simulink library "est_estimator_lib_wState_lib"  (R2016b)
settings: Solver=ode45  StartTime=0.0  StopTime=10.0  RelTol=1e-3  EnableMultiTasking=on
values from neighbouring files (symbols this model uses):
  ase_accel_fixed_bias = single([0 0 0])    [ase_augmented_state_estimator_init.m]    (also in ase_hw_data_test.m = single([-0.1425    0.0852   -9.8201]))
  ase_gyro_fixed_bias = single([0 0 0])    [ase_augmented_state_estimator_init.m]    (also in ase_hw_data_test.m = single(1e-3 * [-1.0787    0.00   0.4470]))
  ase_ml_num_features = Simulink.Parameter(int32(50))    [ase_augmented_state_estimator_init.m]
  ase_of_num_aug = Simulink.Parameter(int32(16))    [ase_augmented_state_estimator_init.m]
  ase_of_num_features = Simulink.Parameter(int32(50))    [ase_augmented_state_estimator_init.m]
  ase_ts = astrobee_fsw_step_size    [ase_augmented_state_estimator_init.m]
undefined symbols (not defined in the file or in its folder): astrobee_fsw_step_size, fam_impeller_speeds, tun_abp_quat_body2imu, tun_ase_gravity_accel, tun_ase_gravity_removal, tun_grav_hp_den, tun_grav_hp_enable_f, tun_grav_hp_num, tun_ic_cov_pos, tun_ic_cov_quat
libraries: simulink x10, math_utils x3, delay_ic_lib x1, camera_update_lib x1, output_prep_lib x1, predictor_lib x1, state_manager_lib x1
settings Model: Creator=jfusco1  LastModifiedBy=jfusco1
settings DataIOCC: LimitDataPoints=on  SaveFormat=Array
settings OptimizationCC: LifeSpan=inf
settings DebuggingCC: AllowSymbolicDim=off  SFUnexpectedBacktrackingDiag=warning  SFNoUnconditionalDefaultTransitionDiag=warning  SFExecutionAtInitializationDiag=none
settings HardwareCC: ProdBitPerPointer=32  ProdBitPerSizeT=32  ProdBitPerPtrDiffT=32  ProdLargestAtomicFloat=None  ProdIntDivRoundTo=Undefined  ProdEndianess=Unspecified  ProdWordSize=32  ProdHWDeviceType=32-bit Generic
settings ModelReferenceCC: PropagateSignalLabelsOutOfModel=off
settings GRTTargetCC: TargetLangStandard=C89/C90 (ANSI)  GeneratePreprocessorConditionals=Disable all
settings ConfigComp: CovMetricSettings=dw  CovHtmlReporting=on  CovSaveCumulativeToWorkspaceVar=on  CovSaveSingleToWorkspaceVar=on  CovExternalEMLEnable=off

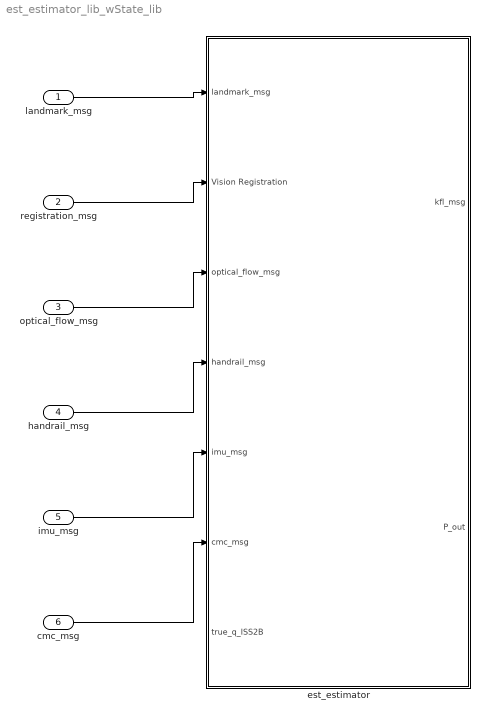
== system est_estimator_lib_wState_lib ==
  landmark_msg : Inport  OutDataTypeStr=Bus: cvs_landmark_msg
  registration_msg : Inport  Port=2  OutDataTypeStr=Bus: cvs_registration_pulse
  optical_flow_msg : Inport  Port=3  OutDataTypeStr=Bus: cvs_optical_flow_msg
  handrail_msg : Inport  Port=4  OutDataTypeStr=Bus: cvs_handrail_msg
  imu_msg : Inport  Port=5  OutDataTypeStr=Bus: imu_msg
  cmc_msg : Inport  Port=6  OutDataTypeStr=Bus: cmc_msg
  est_estimator : Subsystem  TreatAsAtomicUnit=on  SystemSampleTime=ase_ts
  wires:
  landmark_msg/1 -> est_estimator/1(landmark_msg)
  registration_msg/1 -> est_estimator/2(Vision Registration)
  optical_flow_msg/1 -> est_estimator/3(optical_flow_msg)
  handrail_msg/1 -> est_estimator/4(handrail_msg)
  imu_msg/1 -> est_estimator/5(imu_msg)
  cmc_msg/1 -> est_estimator/6(cmc_msg)

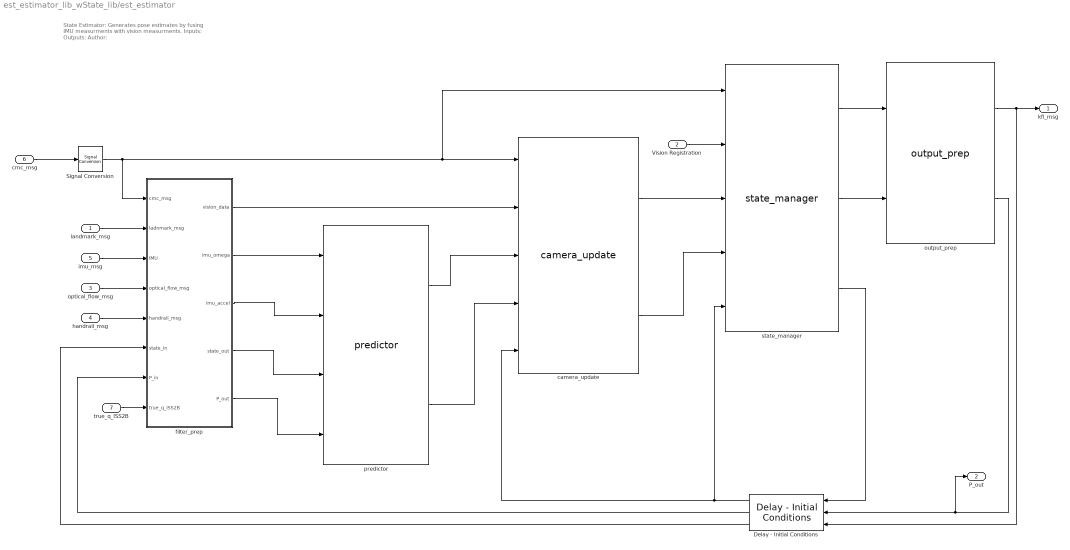
== system est_estimator_lib_wState_lib/est_estimator ==
  note: State Estimator:
      | Generates pose estimates by fusing IMU measurments with vision measurments.
      |
      | Inputs:
      |
      | Outputs:
      |
      | Author:
  landmark_msg : Inport  OutDataTypeStr=Bus: cvs_landmark_msg
  Vision Registration : Inport  Port=2  OutDataTypeStr=Bus: cvs_registration_pulse
  optical_flow_msg : Inport  Port=3  OutDataTypeStr=Bus: cvs_optical_flow_msg
  handrail_msg : Inport  Port=4
  imu_msg : Inport  Port=5  OutDataTypeStr=Bus: imu_msg
  cmc_msg : Inport  Port=6  OutDataTypeStr=Bus: cmc_msg
  true_q_ISS2B : Inport  Port=7
  Delay - Initial Conditions : delay_ic_lib/Delay - Initial Conditions
  Signal Conversion : SignalConversion  OverrideOpt=on
  camera_update : camera_update_lib/camera_update
  filter_prep : Subsystem
  output_prep : output_prep_lib/output_prep
  predictor : predictor_lib/predictor
  state_manager : state_manager_lib/state_manager
  kfl_msg : Outport  OutDataTypeStr=Bus: kfl_msg
  P_out : Outport  Port=2
  wires:
  true_q_ISS2B/1 -> filter_prep/8(true_q_ISS2B)
  filter_prep/5(P_out) -> predictor/4
  Signal Conversion/1 -> state_manager/1, camera_update/1, filter_prep/1(cmc_msg)
  landmark_msg/1 -> filter_prep/2(ladnmark_msg)
  imu_msg/1 -> filter_prep/3(IMU)
  optical_flow_msg/1 -> filter_prep/4(optical_flow_msg)
  handrail_msg/1 -> filter_prep/5(handrail_msg)
  filter_prep/1(vision_data) -> camera_update/2
  predictor/1 -> camera_update/3
  predictor/2 -> camera_update/4
  Vision Registration/1 -> state_manager/2
  camera_update/1 -> state_manager/3
  camera_update/2 -> state_manager/4
  filter_prep/4(state_out) -> predictor/3
  Delay - Initial Conditions/3 -> filter_prep/6(state_in)
  Delay - Initial Conditions/1 -> camera_update/5, state_manager/5
  state_manager/3 -> Delay - Initial Conditions/1
  Delay - Initial Conditions/2 -> filter_prep/7(P_in)
  output_prep/1 -> kfl_msg/1, Delay - Initial Conditions/3
  output_prep/2 -> P_out/1, Delay - Initial Conditions/2
  state_manager/1 -> output_prep/1
  state_manager/2 -> output_prep/2
  filter_prep/3(imu_accel) -> predictor/2
  filter_prep/2(imu_omega) -> predictor/1
  cmc_msg/1 -> Signal Conversion/1

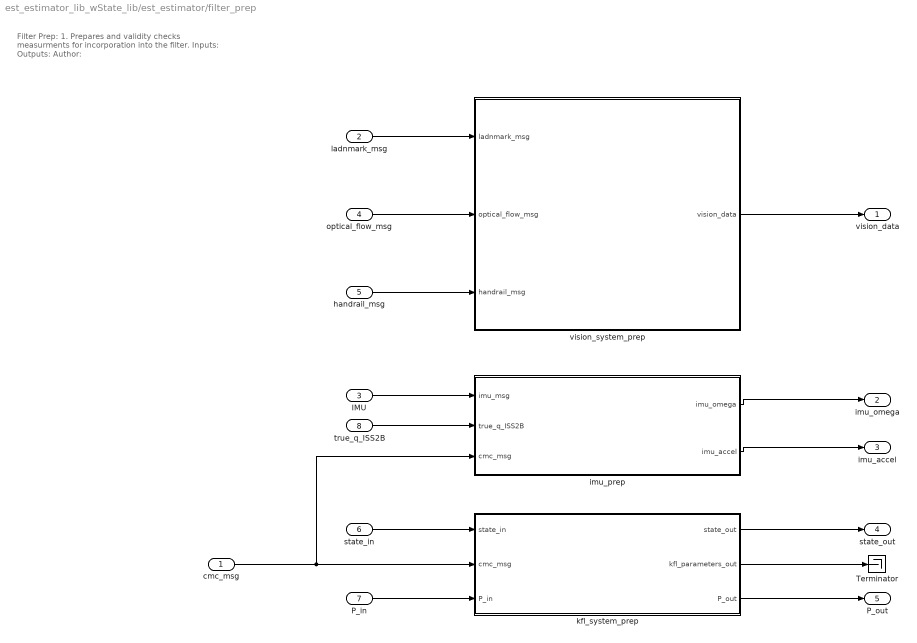
== system est_estimator_lib_wState_lib/est_estimator/filter_prep ==
  note: Filter Prep:
      | 1. Prepares and validity checks measurments for incorporation into the filter.
      |
      | Inputs:
      |
      | Outputs:
      |
      | Author:
  cmc_msg : Inport
  ladnmark_msg : Inport  Port=2  OutDataTypeStr=Bus: cvs_landmark_msg
  IMU : Inport  Port=3  OutDataTypeStr=Bus: imu_msg
  optical_flow_msg : Inport  Port=4  OutDataTypeStr=Bus: cvs_optical_flow_msg
  handrail_msg : Inport  Port=5
  state_in : Inport  Port=6
  P_in : Inport  Port=7
  true_q_ISS2B : Inport  Port=8
  Terminator : Terminator
  imu_prep : Subsystem
  kfl_system_prep : Subsystem
  vision_system_prep : Subsystem
  vision_data : Outport
  imu_omega : Outport  Port=2
  imu_accel : Outport  Port=3
  state_out : Outport  Port=4
  P_out : Outport  Port=5
  wires:
  IMU/1 -> imu_prep/1(imu_msg)
  imu_prep/1(imu_omega) -> imu_omega/1
  imu_prep/2(imu_accel) -> imu_accel/1
  ladnmark_msg/1 -> vision_system_prep/1(ladnmark_msg)
  optical_flow_msg/1 -> vision_system_prep/2(optical_flow_msg)
  handrail_msg/1 -> vision_system_prep/3(handrail_msg)
  vision_system_prep/1(vision_data) -> vision_data/1
  state_in/1 -> kfl_system_prep/1(state_in)
  kfl_system_prep/1(state_out) -> state_out/1
  cmc_msg/1 -> imu_prep/3(cmc_msg), kfl_system_prep/2(cmc_msg)
  P_in/1 -> kfl_system_prep/3(P_in)
  kfl_system_prep/3(P_out) -> P_out/1
  kfl_system_prep/2(kfl_parameters_out) -> Terminator/1
  true_q_ISS2B/1 -> imu_prep/2(true_q_ISS2B)

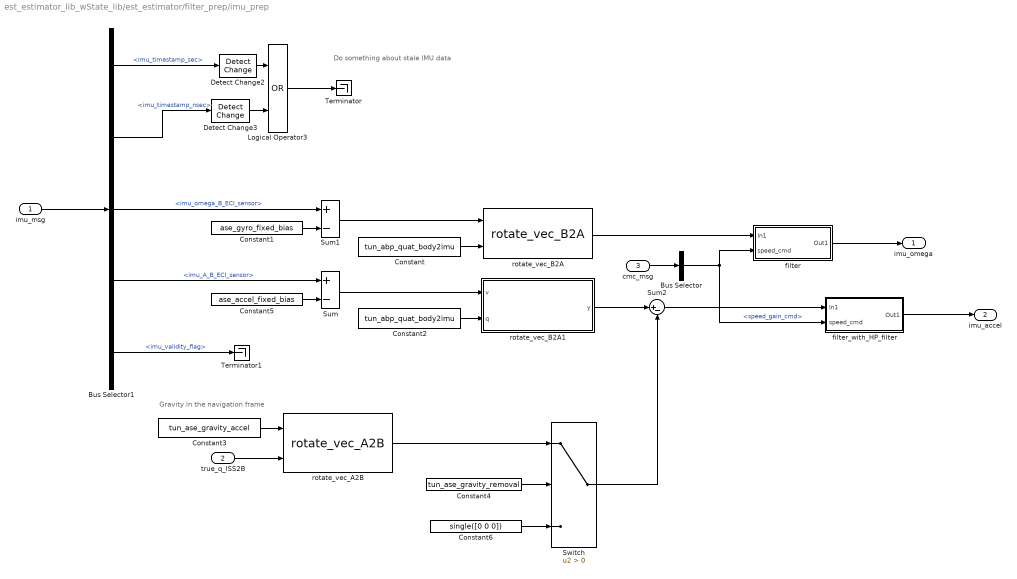
== system est_estimator_lib_wState_lib/est_estimator/filter_prep/imu_prep ==
  note: Do something about stale IMU data
  note: Gravity in the navigation frame
  imu_msg : Inport
  true_q_ISS2B : Inport  Port=2
  cmc_msg : Inport  Port=3  OutDataTypeStr=Bus: cmc_msg
  Bus Selector : BusSelector  OutputSignals=speed_gain_cmd
  Bus Selector1 : BusSelector  OutputSignals=imu_timestamp_sec,imu_timestamp_nsec,imu_omega_B_ECI_sensor,imu_A_B_ECI_sensor,imu_validity_flag
  Constant : Constant  Value=tun_abp_quat_body2imu
  Constant1 : Constant  Value=ase_gyro_fixed_bias
  Constant2 : Constant  Value=tun_abp_quat_body2imu
  Constant3 : Constant  Value=tun_ase_gravity_accel
  Constant4 : Constant  Value=tun_ase_gravity_removal
  Constant5 : Constant  Value=ase_accel_fixed_bias
  Constant6 : Constant  Value=single([0 0 0])
  Detect Change2 : simulink/Logic and Bit Operations/Detect Change  vinit=0  InputProcessing=Inherited  OutDataTypeStr=boolean
  Detect Change3 : simulink/Logic and Bit Operations/Detect Change  vinit=0  InputProcessing=Inherited  OutDataTypeStr=boolean
  Logical Operator3 : Logic  Operator=OR  AllPortsSameDT=off  OutDataTypeStr=boolean
  Sum : Sum  Inputs=+-
  Sum1 : Sum  Inputs=+-
  Sum2 : Sum  Inputs=|+-
  Switch : Switch  Criteria=u2 > Threshold
  Terminator : Terminator
  Terminator1 : Terminator
  filter : Subsystem  TreatAsAtomicUnit=on
  filter_with_HP_filter : Subsystem
  rotate_vec_A2B : math_utils/rotate_vec_A2B  SystemSampleTime=-1
  rotate_vec_B2A : math_utils/rotate_vec_B2A  SystemSampleTime=-1
  rotate_vec_B2A1 : Subsystem
      mask Display:
      | disp('Rotate Vector\n\n')
      | disp('B to A');
  imu_omega : Outport
  imu_accel : Outport  Port=2
  wires:
  imu_msg/1 -> Bus Selector1/1
  Detect Change2/1 -> Logical Operator3/1
  Detect Change3/1 -> Logical Operator3/2
  Bus Selector1/1 -> Detect Change2/1  "<imu_timestamp_sec>"
  Bus Selector1/2 -> Detect Change3/1  "<imu_timestamp_nsec>"
  Logical Operator3/1 -> Terminator/1
  Bus Selector1/5 -> Terminator1/1  "<imu_validity_flag>"
  Bus Selector1/3 -> Sum1/1  "<imu_omega_B_ECI_sensor>"
  Bus Selector1/4 -> Sum/1  "<imu_A_B_ECI_sensor>"
  Constant5/1 -> Sum/2
  Constant1/1 -> Sum1/2
  Constant/1 -> rotate_vec_B2A/2
  Constant2/1 -> rotate_vec_B2A1/2(q)
  Sum1/1 -> rotate_vec_B2A/1
  Sum/1 -> rotate_vec_B2A1/1(v)
  filter_with_HP_filter/1(Out1) -> imu_accel/1
  true_q_ISS2B/1 -> rotate_vec_A2B/2
  Constant3/1 -> rotate_vec_A2B/1
  Constant4/1 -> Switch/2
  rotate_vec_A2B/1 -> Switch/1
  Constant6/1 -> Switch/3
  rotate_vec_B2A1/1(y) -> Sum2/1
  Sum2/1 -> filter_with_HP_filter/1(In1)
  Switch/1 -> Sum2/2
  cmc_msg/1 -> Bus Selector/1
  Bus Selector/1 -> filter/2(speed_cmd), filter_with_HP_filter/2(speed_cmd)  "<speed_gain_cmd>"
  rotate_vec_B2A/1 -> filter/1(In1)
  filter/1(Out1) -> imu_omega/1

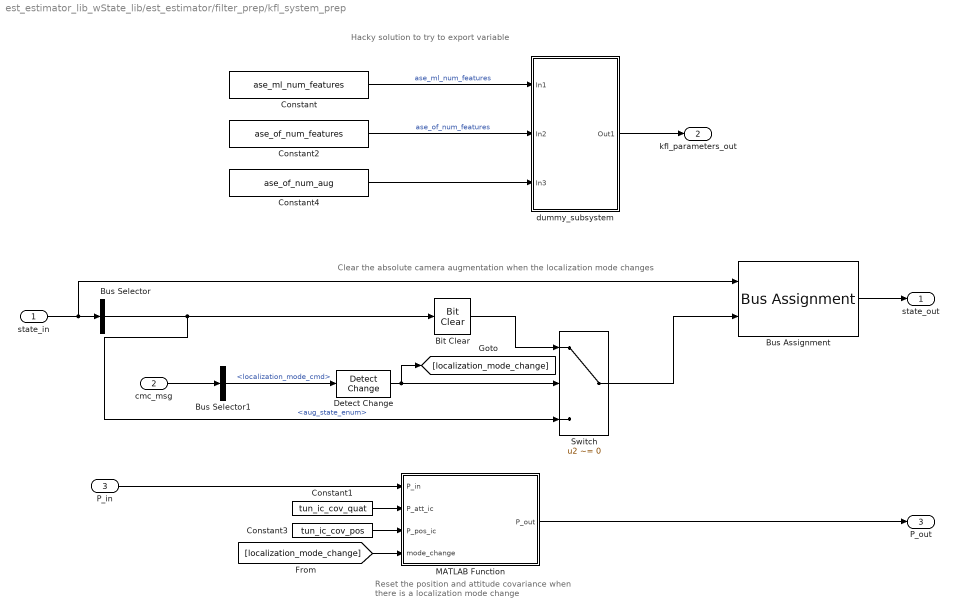
== system est_estimator_lib_wState_lib/est_estimator/filter_prep/kfl_system_prep ==
  note: Clear the absolute camera augmentation when the localization mode changes
  note: Reset the position and attitude covariance when
      | there is a localization mode change
  note: Hacky solution to try to export variable
  state_in : Inport
  cmc_msg : Inport  Port=2
  P_in : Inport  Port=3
  Bit Clear : simulink/Logic and Bit Operations/Bit Clear  iBit=0
  Bus Assignment : BusAssignment  AssignedSignals=aug_state_enum
  Bus Selector : BusSelector  OutputSignals=aug_state_enum
  Bus Selector1 : BusSelector  OutputSignals=localization_mode_cmd
  Constant : Constant  Value=ase_ml_num_features
  Constant1 : Constant  Value=tun_ic_cov_quat
  Constant2 : Constant  Value=ase_of_num_features
  Constant3 : Constant  Value=tun_ic_cov_pos
  Constant4 : Constant  Value=ase_of_num_aug
  Detect Change : simulink/Logic and Bit Operations/Detect Change  vinit=0  InputProcessing=Inherited  OutDataTypeStr=boolean
  MATLAB Function : MATLAB Function  TreatAsAtomicUnit=on
  Switch : Switch  Criteria=u2 ~= 0
  dummy_subsystem : Subsystem  TreatAsAtomicUnit=on
  state_out : Outport
  kfl_parameters_out : Outport  Port=2
  P_out : Outport  Port=3
  wires:
  state_in/1 -> Bus Assignment/1, Bus Selector/1
  cmc_msg/1 -> Bus Selector1/1
  Bus Selector1/1 -> Detect Change/1  "<localization_mode_cmd>"
  Bus Selector/1 -> Switch/3, Bit Clear/1  "<aug_state_enum>"
  Detect Change/1 -> [localization_mode_change], Switch/2
  Bit Clear/1 -> Switch/1
  Switch/1 -> Bus Assignment/2
  Bus Assignment/1 -> state_out/1
  Constant1/1 -> MATLAB Function/2(P_att_ic)
  Constant3/1 -> MATLAB Function/3(P_pos_ic)
  [localization_mode_change] -> MATLAB Function/4(mode_change)
  P_in/1 -> MATLAB Function/1(P_in)
  MATLAB Function/1(P_out) -> P_out/1
  Constant2/1 -> dummy_subsystem/2(In2)  "ase_of_num_features"
  Constant/1 -> dummy_subsystem/1(In1)  "ase_ml_num_features"
  dummy_subsystem/1(Out1) -> kfl_parameters_out/1
  Constant4/1 -> dummy_subsystem/3(In3)

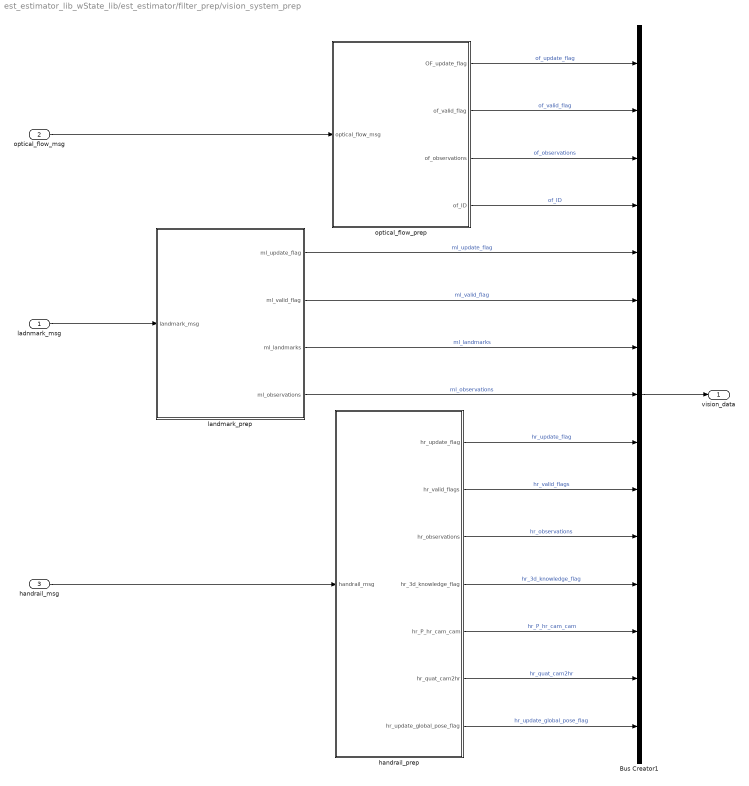
== system est_estimator_lib_wState_lib/est_estimator/filter_prep/vision_system_prep ==
  ladnmark_msg : Inport  OutDataTypeStr=Bus: cvs_landmark_msg
  optical_flow_msg : Inport  Port=2  OutDataTypeStr=Bus: cvs_optical_flow_msg
  handrail_msg : Inport  Port=3
  Bus Creator1 : BusCreator  Inputs=15
  handrail_prep : Subsystem
  landmark_prep : Subsystem
  optical_flow_prep : Subsystem
  vision_data : Outport
  wires:
  handrail_prep/4(hr_3d_knowledge_flag) -> Bus Creator1/12  "hr_3d_knowledge_flag"
  ladnmark_msg/1 -> landmark_prep/1(landmark_msg)
  optical_flow_msg/1 -> optical_flow_prep/1(optical_flow_msg)
  optical_flow_prep/3(of_observations) -> Bus Creator1/3  "of_observations"
  optical_flow_prep/1(OF_update_flag) -> Bus Creator1/1  "of_update_flag"
  Bus Creator1/1 -> vision_data/1
  handrail_prep/2(hr_valid_flags) -> Bus Creator1/10  "hr_valid_flags"
  handrail_prep/1(hr_update_flag) -> Bus Creator1/9  "hr_update_flag"
  handrail_msg/1 -> handrail_prep/1(handrail_msg)
  landmark_prep/1(ml_update_flag) -> Bus Creator1/5  "ml_update_flag"
  optical_flow_prep/2(of_valid_flag) -> Bus Creator1/2  "of_valid_flag"
  optical_flow_prep/4(of_ID) -> Bus Creator1/4  "of_ID"
  landmark_prep/2(ml_valid_flag) -> Bus Creator1/6  "ml_valid_flag"
  landmark_prep/3(ml_landmarks) -> Bus Creator1/7  "ml_landmarks"
  landmark_prep/4(ml_observations) -> Bus Creator1/8  "ml_observations"
  handrail_prep/3(hr_observations) -> Bus Creator1/11  "hr_observations"
  handrail_prep/7(hr_update_global_pose_flag) -> Bus Creator1/15  "hr_update_global_pose_flag"
  handrail_prep/5(hr_P_hr_cam_cam) -> Bus Creator1/13  "hr_P_hr_cam_cam"
  handrail_prep/6(hr_quat_cam2hr) -> Bus Creator1/14  "hr_quat_cam2hr"

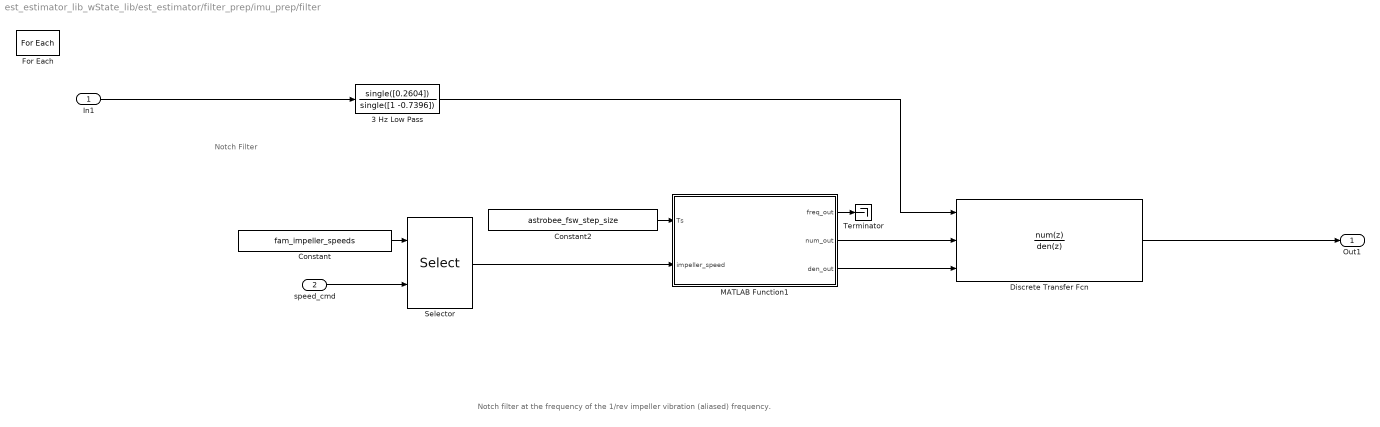
== system est_estimator_lib_wState_lib/est_estimator/filter_prep/imu_prep/filter ==
  note: Notch filter at the frequency of the 1/rev impeller vibration (aliased) frequency.
  note: Notch Filter
  In1 : Inport  Partition=on  PartitionDimension=1  PartitionWidth=1
  speed_cmd : Inport  Port=2
  3 Hz Low Pass : DiscreteTransferFcn  Numerator=single([0.2604])  Denominator=single([1 -0.7396])  SampleTime=1/62.5
  Constant : Constant  Value=fam_impeller_speeds
  Constant2 : Constant  Value=astrobee_fsw_step_size
  Discrete Transfer Fcn : DiscreteTransferFcn  NumeratorSource=Input port  Numerator=[1.817 3.554 1.817]  DenominatorSource=Input port  Denominator=[2 3.554 1.633]  SampleTime=astrobee_fsw_step_size  a0EqualsOne=on
      settings: InputPortMap=u0,p1,p3
  For Each : ForEach  DisableCoverage=on  IndexMode=One-based
  MATLAB Function1 : MATLAB Function  TreatAsAtomicUnit=on
  Selector : Selector  InputPortWidth=3  IndexOptions=Index vector (port)  Indices=[1 3]  OutputSizes=1
  Terminator : Terminator
  Out1 : Outport  ConcatenationDimension=1
  wires:
  In1/1 -> 3 Hz Low Pass/1
  3 Hz Low Pass/1 -> Discrete Transfer Fcn/1
  speed_cmd/1 -> Selector/2
  Constant/1 -> Selector/1
  Selector/1 -> MATLAB Function1/2(impeller_speed)
  MATLAB Function1/1(freq_out) -> Terminator/1
  Constant2/1 -> MATLAB Function1/1(Ts)
  MATLAB Function1/2(num_out) -> Discrete Transfer Fcn/2
  MATLAB Function1/3(den_out) -> Discrete Transfer Fcn/3
  Discrete Transfer Fcn/1 -> Out1/1

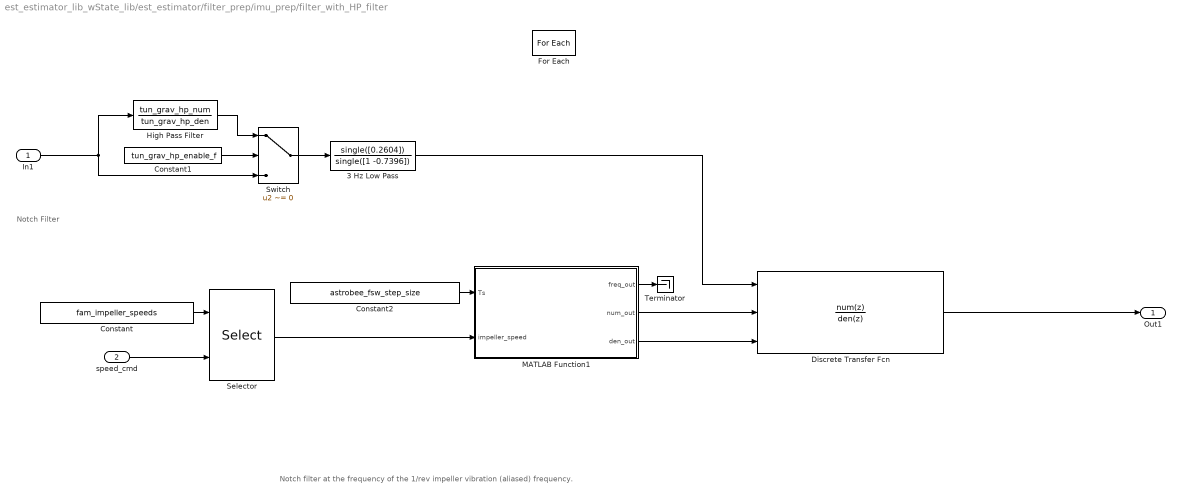
== system est_estimator_lib_wState_lib/est_estimator/filter_prep/imu_prep/filter_with_HP_filter ==
  note: Notch filter at the frequency of the 1/rev impeller vibration (aliased) frequency.
  note: Notch Filter
  In1 : Inport  Partition=on  PartitionDimension=1  PartitionWidth=1
  speed_cmd : Inport  Port=2
  3 Hz Low Pass : DiscreteTransferFcn  Numerator=single([0.2604])  Denominator=single([1 -0.7396])  SampleTime=1/62.5
  Constant : Constant  Value=fam_impeller_speeds
  Constant1 : Constant  Value=tun_grav_hp_enable_f
  Constant2 : Constant  Value=astrobee_fsw_step_size
  Discrete Transfer Fcn : DiscreteTransferFcn  NumeratorSource=Input port  Numerator=[1.817 3.554 1.817]  DenominatorSource=Input port  Denominator=[2 3.554 1.633]  SampleTime=astrobee_fsw_step_size  a0EqualsOne=on
      settings: InputPortMap=u0,p1,p3
  For Each : ForEach  DisableCoverage=on  IndexMode=One-based
  High Pass Filter : DiscreteTransferFcn  Numerator=tun_grav_hp_num  Denominator=tun_grav_hp_den  SampleTime=1/62.5
  MATLAB Function1 : MATLAB Function  TreatAsAtomicUnit=on
  Selector : Selector  InputPortWidth=3  IndexOptions=Index vector (port)  Indices=[1 3]  OutputSizes=1
  Switch : Switch  Criteria=u2 ~= 0
  Terminator : Terminator
  Out1 : Outport  ConcatenationDimension=1
  wires:
  High Pass Filter/1 -> Switch/1
  Constant1/1 -> Switch/2
  Switch/1 -> 3 Hz Low Pass/1
  In1/1 -> High Pass Filter/1, Switch/3
  3 Hz Low Pass/1 -> Discrete Transfer Fcn/1
  speed_cmd/1 -> Selector/2
  Constant/1 -> Selector/1
  Selector/1 -> MATLAB Function1/2(impeller_speed)
  MATLAB Function1/1(freq_out) -> Terminator/1
  Constant2/1 -> MATLAB Function1/1(Ts)
  MATLAB Function1/2(num_out) -> Discrete Transfer Fcn/2
  MATLAB Function1/3(den_out) -> Discrete Transfer Fcn/3
  Discrete Transfer Fcn/1 -> Out1/1

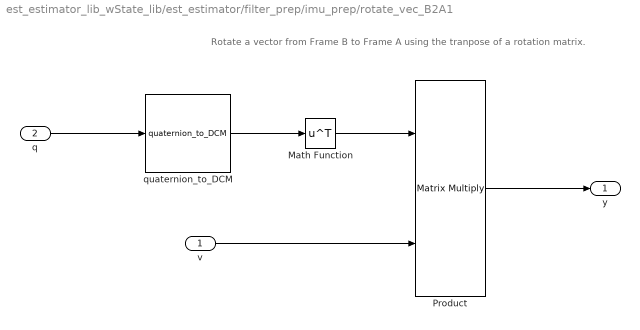
== system est_estimator_lib_wState_lib/est_estimator/filter_prep/imu_prep/rotate_vec_B2A1 ==
  note: Rotate a vector from Frame B to Frame A using the tranpose of a rotation matrix.
  v : Inport
  q : Inport  Port=2
  Math Function : Math  Operator=transpose  SaturateOnIntegerOverflow=on
  Product : Product  Multiplication=Matrix(*)
  quaternion_to_DCM : math_utils/quaternion_to_DCM  SystemSampleTime=-1
  y : Outport
  wires:
  Product/1 -> y/1
  v/1 -> Product/2
  quaternion_to_DCM/1 -> Math Function/1
  q/1 -> quaternion_to_DCM/1
  Math Function/1 -> Product/1

== system est_estimator_lib_wState_lib/est_estimator/filter_prep/kfl_system_prep/dummy_subsystem ==
  In1 : Inport
  In2 : Inport  Port=2
  In3 : Inport  Port=3
  Bus Creator : BusCreator  Inputs=3
  Out1 : Outport
  wires:
  In1/1 -> Bus Creator/1
  In2/1 -> Bus Creator/2
  Bus Creator/1 -> Out1/1
  In3/1 -> Bus Creator/3

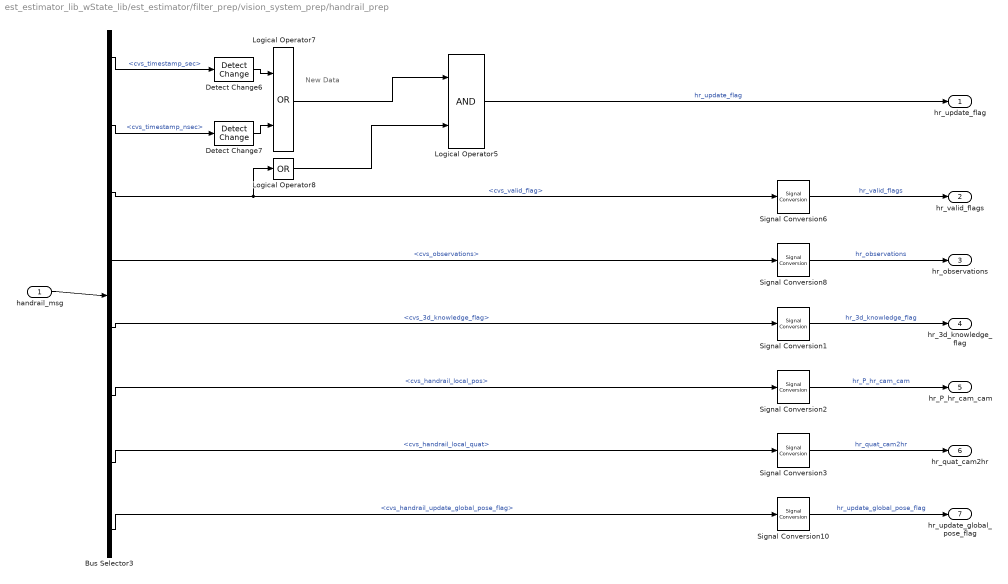
== system est_estimator_lib_wState_lib/est_estimator/filter_prep/vision_system_prep/handrail_prep ==
  note: New Data
  handrail_msg : Inport
  Bus Selector3 : BusSelector  OutputSignals=cvs_timestamp_sec,cvs_timestamp_nsec,cvs_valid_flag,cvs_observations,cvs_3d_knowledge_flag,cvs_handrail_local_pos,cvs_handrail_local_quat,cvs_handrail_update_global_pose_flag
  Detect Change6 : simulink/Logic and Bit Operations/Detect Change  vinit=0  InputProcessing=Inherited  OutDataTypeStr=boolean
  Detect Change7 : simulink/Logic and Bit Operations/Detect Change  vinit=0  InputProcessing=Inherited  OutDataTypeStr=boolean
  Logical Operator5 : Logic  AllPortsSameDT=off  OutDataTypeStr=boolean
  Logical Operator7 : Logic  Operator=OR  AllPortsSameDT=off  OutDataTypeStr=boolean
  Logical Operator8 : Logic  Operator=OR  Inputs=1  AllPortsSameDT=off  OutDataTypeStr=boolean
  Signal Conversion{1..3,6,8,10} (6 alike) : SignalConversion  OverrideOpt=off
  hr_update_flag : Outport
  hr_valid_flags : Outport  Port=2
  hr_observations : Outport  Port=3
  hr_3d_knowledge_flag : Outport  Port=4
  hr_P_hr_cam_cam : Outport  Port=5
  hr_quat_cam2hr : Outport  Port=6
  hr_update_global_pose_flag : Outport  Port=7
  wires:
  Bus Selector3/5 -> Signal Conversion1/1  "<cvs_3d_knowledge_flag>"
  Signal Conversion1/1 -> hr_3d_knowledge_flag/1  "hr_3d_knowledge_flag"
  Bus Selector3/4 -> Signal Conversion8/1  "<cvs_observations>"
  Signal Conversion8/1 -> hr_observations/1  "hr_observations"
  Signal Conversion6/1 -> hr_valid_flags/1  "hr_valid_flags"
  Logical Operator5/1 -> hr_update_flag/1  "hr_update_flag"
  Logical Operator8/1 -> Logical Operator5/2
  Bus Selector3/3 -> Signal Conversion6/1, Logical Operator8/1  "<cvs_valid_flag>"
  Bus Selector3/2 -> Detect Change7/1  "<cvs_timestamp_nsec>"
  Bus Selector3/1 -> Detect Change6/1  "<cvs_timestamp_sec>"
  Detect Change6/1 -> Logical Operator7/1
  Detect Change7/1 -> Logical Operator7/2
  Logical Operator7/1 -> Logical Operator5/1
  handrail_msg/1 -> Bus Selector3/1
  Bus Selector3/6 -> Signal Conversion2/1  "<cvs_handrail_local_pos>"
  Signal Conversion2/1 -> hr_P_hr_cam_cam/1  "hr_P_hr_cam_cam"
  Bus Selector3/7 -> Signal Conversion3/1  "<cvs_handrail_local_quat>"
  Signal Conversion3/1 -> hr_quat_cam2hr/1  "hr_quat_cam2hr"
  Bus Selector3/8 -> Signal Conversion10/1  "<cvs_handrail_update_global_pose_flag>"
  Signal Conversion10/1 -> hr_update_global_pose_flag/1  "hr_update_global_pose_flag"

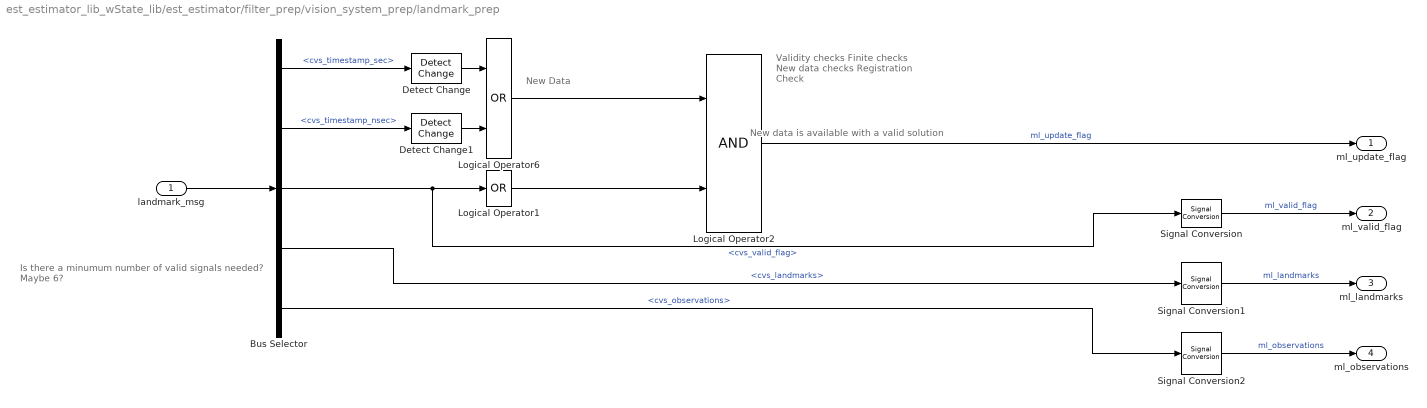
== system est_estimator_lib_wState_lib/est_estimator/filter_prep/vision_system_prep/landmark_prep ==
  note: New Data
  note: New data is available with a valid solution
  note: Validity checks
      | Finite checks
      | New data checks
      | Registration Check
  note: Is there a minumum number of valid signals needed?
      | Maybe 6?
  landmark_msg : Inport
  Bus Selector : BusSelector  OutputSignals=cvs_timestamp_sec,cvs_timestamp_nsec,cvs_valid_flag,cvs_landmarks,cvs_observations
  Detect Change : simulink/Logic and Bit Operations/Detect Change  vinit=0  InputProcessing=Inherited  OutDataTypeStr=boolean
  Detect Change1 : simulink/Logic and Bit Operations/Detect Change  vinit=0  InputProcessing=Inherited  OutDataTypeStr=boolean
  Logical Operator1 : Logic  Operator=OR  Inputs=1  AllPortsSameDT=off  OutDataTypeStr=boolean
  Logical Operator2 : Logic  AllPortsSameDT=off  OutDataTypeStr=boolean
  Logical Operator6 : Logic  Operator=OR  AllPortsSameDT=off  OutDataTypeStr=boolean
  Signal Conversion : SignalConversion  OverrideOpt=off
  Signal Conversion1 : SignalConversion  OverrideOpt=off
  Signal Conversion2 : SignalConversion  OverrideOpt=off
  ml_update_flag : Outport
  ml_valid_flag : Outport  Port=2
  ml_landmarks : Outport  Port=3
  ml_observations : Outport  Port=4
  wires:
  Logical Operator2/1 -> ml_update_flag/1  "ml_update_flag"
  Bus Selector/3 -> Logical Operator1/1, Signal Conversion/1  "<cvs_valid_flag>"
  Logical Operator6/1 -> Logical Operator2/1
  Logical Operator1/1 -> Logical Operator2/2
  landmark_msg/1 -> Bus Selector/1
  Detect Change/1 -> Logical Operator6/1
  Detect Change1/1 -> Logical Operator6/2
  Bus Selector/2 -> Detect Change1/1  "<cvs_timestamp_nsec>"
  Bus Selector/1 -> Detect Change/1  "<cvs_timestamp_sec>"
  Bus Selector/4 -> Signal Conversion1/1  "<cvs_landmarks>"
  Bus Selector/5 -> Signal Conversion2/1  "<cvs_observations>"
  Signal Conversion2/1 -> ml_observations/1  "ml_observations"
  Signal Conversion/1 -> ml_valid_flag/1  "ml_valid_flag"
  Signal Conversion1/1 -> ml_landmarks/1  "ml_landmarks"

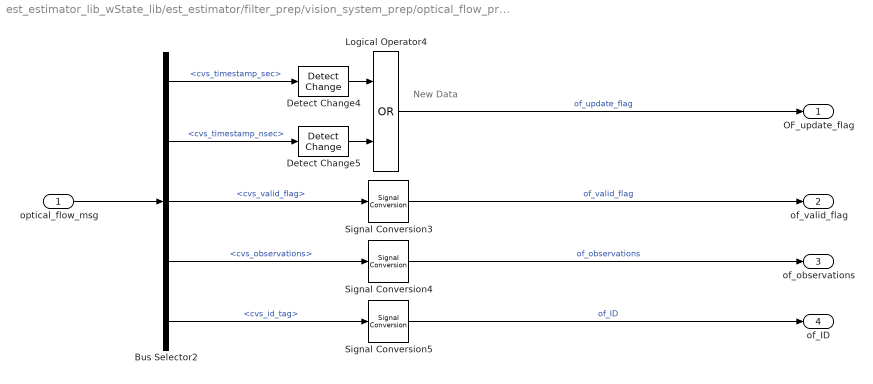
== system est_estimator_lib_wState_lib/est_estimator/filter_prep/vision_system_prep/optical_flow_prep ==
  note: New Data
  optical_flow_msg : Inport
  Bus Selector2 : BusSelector  OutputSignals=cvs_timestamp_sec,cvs_timestamp_nsec,cvs_valid_flag,cvs_observations,cvs_id_tag
  Detect Change4 : simulink/Logic and Bit Operations/Detect Change  vinit=0  InputProcessing=Inherited  OutDataTypeStr=boolean
  Detect Change5 : simulink/Logic and Bit Operations/Detect Change  vinit=0  InputProcessing=Inherited  OutDataTypeStr=boolean
  Logical Operator4 : Logic  Operator=OR  AllPortsSameDT=off  OutDataTypeStr=boolean
  Signal Conversion3 : SignalConversion  OverrideOpt=off
  Signal Conversion4 : SignalConversion  OverrideOpt=off
  Signal Conversion5 : SignalConversion  OverrideOpt=off
  OF_update_flag : Outport
  of_valid_flag : Outport  Port=2
  of_observations : Outport  Port=3
  of_ID : Outport  Port=4
  wires:
  Bus Selector2/2 -> Detect Change5/1  "<cvs_timestamp_nsec>"
  Signal Conversion5/1 -> of_ID/1  "of_ID"
  Signal Conversion4/1 -> of_observations/1  "of_observations"
  Bus Selector2/4 -> Signal Conversion4/1  "<cvs_observations>"
  Logical Operator4/1 -> OF_update_flag/1  "of_update_flag"
  Bus Selector2/3 -> Signal Conversion3/1  "<cvs_valid_flag>"
  Bus Selector2/1 -> Detect Change4/1  "<cvs_timestamp_sec>"
  Detect Change4/1 -> Logical Operator4/1
  Detect Change5/1 -> Logical Operator4/2
  optical_flow_msg/1 -> Bus Selector2/1
  Signal Conversion3/1 -> of_valid_flag/1  "of_valid_flag"
  Bus Selector2/5 -> Signal Conversion5/1  "<cvs_id_tag>"

== matlab function est_estimator_lib_wState_lib/est_estimator/filter_prep/imu_prep/filter/MATLAB Function1 ==
  data: Ts input; freq_out output; impeller_speed input; num_out output; den_out output
function [freq_out, num_out, den_out] = fcn(Ts, impeller_speed)
%#codegen
% Calculate notch filter coefficients, note only executes when the impeller speeds change

% Setup to only run when the impeller_speed changes
persistent y 
persistent num 
persistent den 
persistent prev_impeller_speed


if isempty(prev_impeller_speed)
    prev_impeller_speed = single(-1.0); % No number will be equal to NaN, this will trigger the coefficients to update on the first tick
    y = single(0);
    den = single([0 0 1]);
    num = single([0 0 1]);

end
   

% update_flag = (prev_impeller_speed ~= impeller_speed);
if  prev_impeller_speed ~= impeller_speed
    
    bw = 2*2*pi; % Filter Bandwidth
    Fs = 1/Ts; % Sample frequency, Hz
    Ws = 2*pi*Fs; % Sample frequency, Rad/sec
    Nyquist_W = Ws/2; % Nyquist rate, rad/sec
    
    Aliased_W = abs(Ws*[0:3] - impeller_speed); % Look for the possible aliased frequncies
    
    % Find the actual aliased frequency
    impeller_freq = Aliased_W(find(Aliased_W > 0 & Aliased_W <= Nyquist_W, 1, 'first'));
    
    if ~isempty(impeller_freq)
        y = impeller_freq(1); % Impeller frequency
        Omega_n = pi*y/Nyquist_W; % Normalized frequency
        delta_n = pi*bw/Nyquist_W; % Normalized bandwidth
        
        % Calc coefficients of filter, from:
        % http://onlinelibrary.wiley.com/store/10.1002/mop.23439/asset/23439_ftp.pdf?v=1&t=iyyqfya1&s=b26e8f569108cf78a04dbd5e7edb44f70b9bc3d1
        k1 = -cos(Omega_n); 
        k2 = (1-tan(delta_n/2))/(1+tan(delta_n/2));
        num = [1+k2 2*k1*(1+k2) (k2+1)]/2;
        den = [1 k1*(1+k2) k2];
    else
        
        y = single(0);
        num = single([0 0 1]);
        den = single([0 0 1]);
    end
    
end

prev_impeller_speed = impeller_speed;
freq_out = y;
num_out = num;
den_out = den;

== matlab function est_estimator_lib_wState_lib/est_estimator/filter_prep/kfl_system_prep/MATLAB Function ==
  data: P_in input; P_out output; P_att_ic input; P_pos_ic input; mode_change input
function P_out = fcn(P_in, P_att_ic, P_pos_ic, mode_change)
%#codegen

 P_out = P_in;

if mode_change
   % Quat covariance is 1:3, Pos covariance is 13:15
    P_out(1:3,:) = 0;
    P_out(:,1:3) = 0;
    P_out(1:3,1:3) = diag(repmat(P_att_ic,3,1));
    
    P_out(13:15,:) = 0;
    P_out(:,13:15) = 0;
    P_out(13:15,13:15) = diag(repmat(P_pos_ic,3,1));

end

== matlab function est_estimator_lib_wState_lib/est_estimator/filter_prep/imu_prep/filter_with_HP_filter/MATLAB Function1 ==
  data: Ts input; freq_out output; impeller_speed input; num_out output; den_out output
function [freq_out, num_out, den_out] = fcn(Ts, impeller_speed)
%#codegen
% Calculate notch filter coefficients, note only executes when the impeller speeds change

% Setup to only run when the impeller_speed changes
persistent y 
persistent num 
persistent den 
persistent prev_impeller_speed


if isempty(prev_impeller_speed)
    prev_impeller_speed = single(-1.0); % No number will be equal to NaN, this will trigger the coefficients to update on the first tick
    y = single(0);
    den = single([0 0 1]);
    num = single([0 0 1]);

end
   

% update_flag = (prev_impeller_speed ~= impeller_speed);
if  prev_impeller_speed ~= impeller_speed
    
    bw = 2*2*pi; % Filter Bandwidth
    Fs = 1/Ts; % Sample frequency, Hz
    Ws = 2*pi*Fs; % Sample frequency, Rad/sec
    Nyquist_W = Ws/2; % Nyquist rate, rad/sec
    
    Aliased_W = abs(Ws*[0:3] - impeller_speed); % Look for the possible aliased frequncies
    
    % Find the actual aliased frequency
    impeller_freq = Aliased_W(find(Aliased_W > 0 & Aliased_W <= Nyquist_W, 1, 'first'));
    
    if ~isempty(impeller_freq)
        y = impeller_freq(1); % Impeller frequency
        Omega_n = pi*y/Nyquist_W; % Normalized frequency
        delta_n = pi*bw/Nyquist_W; % Normalized bandwidth
        
        % Calc coefficients of filter, from:
        % http://onlinelibrary.wiley.com/store/10.1002/mop.23439/asset/23439_ftp.pdf?v=1&t=iyyqfya1&s=b26e8f569108cf78a04dbd5e7edb44f70b9bc3d1
        k1 = -cos(Omega_n); 
        k2 = (1-tan(delta_n/2))/(1+tan(delta_n/2));
        num = [1+k2 2*k1*(1+k2) (k2+1)]/2;
        den = [1 k1*(1+k2) k2];
    else
        
        y = single(0);
        num = single([0 0 1]);
        den = single([0 0 1]);
    end
    
end

prev_impeller_speed = impeller_speed;
freq_out = y;
num_out = num;
den_out = den;
